simulink model "modelZSBmex"  (Simulink 8.3)
settings: Solver=ode4  StartTime=0.0  StopTime=0.2  FixedStep=0.01  RelTol=1e-3
settings Model: Creator=Chan Hwaiwing  LastModifiedBy=shubo
settings DataIOCC: SignalLoggingSaveFormat=Dataset
settings OptimizationCC: OptimizeModelRefInitCode=on  LifeSpan=1
settings DebuggingCC: UnderspecifiedInitializationDetection=Simplified  MergeDetectMultiDrivingBlocksExec=error  FrameProcessingCompatibilityMsg=error  StateNameClashWarn=none
settings RTWCC: SystemTargetFile=ert.tlc  TemplateMakefile=ert_default_tmf  Description=Embedded Coder  ProcessScript=ert_make_rtw_hook  BuildConfiguration=Faster Runs
settings CodeAppCC: IgnoreCustomStorageClasses=off
settings ERTTargetCC: MultiwordLength=2048  GenerateSampleERTMain=on  SupportNonFinite=off  SupportComplex=off  SupportContinuousTime=on  ERTCustomFileTemplate=example_file_process.tlc  ConvertIfToSwitch=off  SuppressUnreachableDefaultCases=off
settings ConfigComp: CovCompData="CovMetricSettings\t  dw"  CovFilter=CovHTMLOptions  CovHtmlReporting=on  CovSaveCumulativeToWorkspaceVar=on  CovSaveSingleToWorkspaceVar=on  CovModelRefExcluded="CovExternalEMLEnable\t  off"  CovSFcnEnable=off

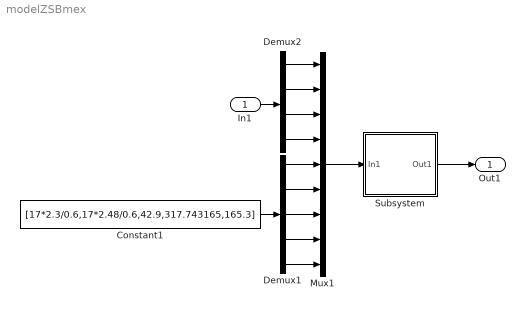
== system modelZSBmex ==
  In1 : Inport
  Constant1 : Constant  Value=[17*2.3/0.6,17*2.48/0.6,42.9,317.743165,165.3]
  Demux1 : Demux  Outputs=5
  Demux2 : Demux
  Mux1 : Mux  Inputs=9
  Subsystem : Subsystem
  Out1 : Outport
  wires:
  Subsystem/1(Out1) -> Out1/1
  Demux2/2 -> Mux1/2
  Demux2/4 -> Mux1/4
  Demux2/3 -> Mux1/3
  Demux2/1 -> Mux1/1
  Mux1/1 -> Subsystem/1(In1)
  In1/1 -> Demux2/1
  Constant1/1 -> Demux1/1
  Demux1/5 -> Mux1/9
  Demux1/2 -> Mux1/6
  Demux1/3 -> Mux1/7
  Demux1/4 -> Mux1/8
  Demux1/1 -> Mux1/5

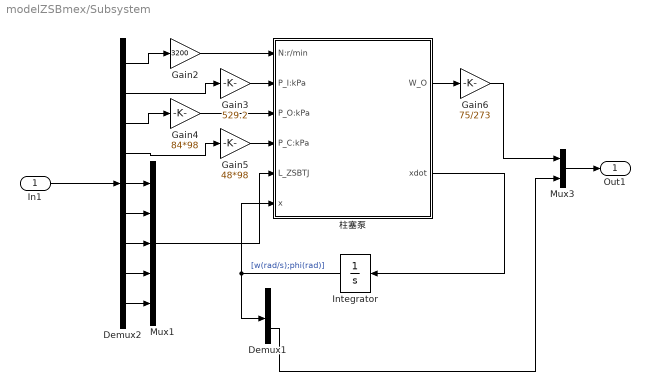
== system modelZSBmex/Subsystem ==
  In1 : Inport
  Demux1 : Demux  Outputs=2
  Demux2 : Demux  Outputs=9
  Gain2 : Gain  Gain=3200
  Gain3 : Gain  Gain=529.2
  Gain4 : Gain  Gain=84*98
  Gain5 : Gain  Gain=48*98
  Gain6 : Gain  Gain=75/273
  Integrator : Integrator  LimitOutput=on  UpperSaturationLimit=[999999 14.8/180*pi]  LowerSaturationLimit=[-999999 -0/180*pi ]
  Mux1 : Mux  Inputs=5
  Mux3 : Mux  Inputs=2
  柱塞泵 : Subsystem  AncestorBlock=HMMtoolbox/泵类/ZSB  mask(柱塞泵){L_ZSBHX=15, D_ZSBZS=48*2, A_ZSBZS=23.8*23.8*pi/4, RHO=780, ETA_V=0.95, M_ZS=0.1006, Z_ZSBZS=7, BETA_ZSBZS=12/180*pi, A_ZSBTJ=[pi*(33.26^2-17^2)/4, pi*(33.26^2-19.8^2)/4], L_ZSBTJ=[45 70 44 319 167], k=((1421-754.6)/((139.7-101.9)-(139.7-119.6))+(1754-1313)/((158-96.8)-(158-114.6)))*1e3*0.4, BETA_ZSBSD=6.97/180*pi, L_x0=139.7+85, J_ZSBXP=0.34*0.05, KD=7.65*0.5}
      mask prompts: L_ZSBHX "L_HX(等效滑靴厚度mm)"; D_ZSBZS "D_ZS(柱塞轴线在缸体的分布圆直径mm)"; A_ZSBZS "A_ZS(柱塞截面面积mm^2)"; RHO "RHO(标准状态下，油液密度kg/m^3)"; ETA_V "ETA_V(容积效率)"; M_ZS "M_ZS(柱塞质量)"; Z_ZSBZS "Z_ZS(柱塞数量)"; BETA_ZSBZS "BETA_ZS(柱塞安装角rad)"; A_ZSBTJ "A_TJ(面积参数向量mm^2)"; L_ZSBTJ "L_TJ(距离参数向量mm)"; k "k(弹簧弹性模量N/m)"; BETA_ZSBSD "BETA_SD(随动活塞安装角rad)"; L_x0 "L_x0(随动活塞初始位置mm)"; J_ZSBXP "J_XP(斜盘绕斜盘轴的转动惯量kg·m^2)"; KD "KD(斜盘转动阻力系数N·m·s/rad)"
      mask DialogControl DescTextVar Prompt: 填入相关参数
  Out1 : Outport
  wires:
  Gain2/1 -> 柱塞泵/1(N:r/min)
  Demux2/3 -> Gain4/1
  Mux3/1 -> Out1/1
  Gain3/1 -> 柱塞泵/2(P_I:kPa)
  In1/1 -> Demux2/1
  Integrator/1 -> Demux1/1, 柱塞泵/6(x)  "[w(rad/s);phi(rad)]"
  Demux2/2 -> Gain3/1
  Demux2/4 -> Gain5/1
  Demux2/1 -> Gain2/1
  柱塞泵/2(xdot) -> Integrator/1
  Mux1/1 -> 柱塞泵/5(L_ZSBTJ)
  柱塞泵/1(W_O) -> Gain6/1
  Gain6/1 -> Mux3/1
  Demux1/2 -> Mux3/2
  Gain4/1 -> 柱塞泵/3(P_O:kPa)
  Gain5/1 -> 柱塞泵/4(P_C:kPa)
  Demux2/5 -> Mux1/1
  Demux2/6 -> Mux1/2
  Demux2/9 -> Mux1/5
  Demux2/8 -> Mux1/4
  Demux2/7 -> Mux1/3

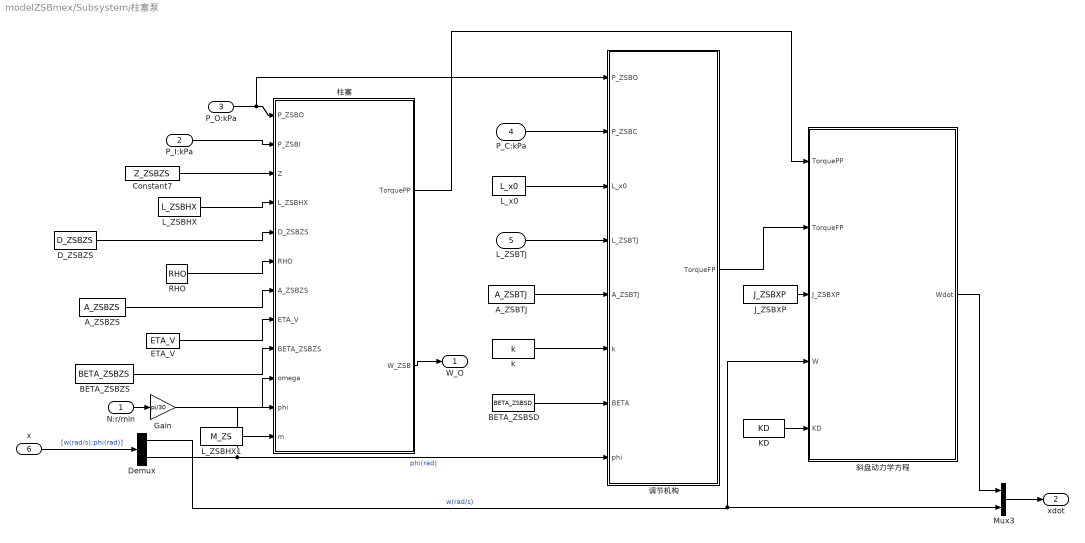
== system modelZSBmex/Subsystem/柱塞泵 ==
  N:r/min : Inport
  P_I:kPa : Inport  Port=2
  P_O:kPa : Inport  Port=3
  P_C:kPa : Inport  Port=4
  L_ZSBTJ : Inport  Port=5
  x : Inport  Port=6
  A_ZSBTJ : Constant  Value=A_ZSBTJ
  A_ZSBZS : Constant  Value=A_ZSBZS
  BETA_ZSBSD : Constant  Value=BETA_ZSBSD
  BETA_ZSBZS : Constant  Value=BETA_ZSBZS
  Constant7 : Constant  Value=Z_ZSBZS
  D_ZSBZS : Constant  Value=D_ZSBZS
  Demux : Demux  Outputs=2
  ETA_V : Constant  Value=ETA_V
  Gain : Gain  Gain=pi/30
  J_ZSBXP : Constant  Value=J_ZSBXP
  KD : Constant  Value=KD
  L_ZSBHX : Constant  Value=L_ZSBHX
  L_ZSBHX1 : Constant  Value=M_ZS
  L_x0 : Constant  Value=L_x0
  Mux3 : Mux  Inputs=2
  RHO : Constant  Value=RHO
  k : Constant  Value=k
  斜盘动力学方程 : MATLAB Function  TreatAsAtomicUnit=on
  柱塞 : MATLAB Function  TreatAsAtomicUnit=on
  调节机构 : MATLAB Function  TreatAsAtomicUnit=on
  W_O : Outport
  xdot : Outport  Port=2
  wires:
  x/1 -> Demux/1  "[w(rad/s);phi(rad)]"
  斜盘动力学方程/1(Wdot) -> Mux3/1
  Mux3/1 -> xdot/1
  J_ZSBXP/1 -> 斜盘动力学方程/3(J_ZSBXP)
  A_ZSBTJ/1 -> 调节机构/5(A_ZSBTJ)
  BETA_ZSBZS/1 -> 柱塞/9(BETA_ZSBZS)
  ETA_V/1 -> 柱塞/8(ETA_V)
  D_ZSBZS/1 -> 柱塞/5(D_ZSBZS)
  Demux/1 -> 斜盘动力学方程/4(W), Mux3/2  "w(rad/s)"
  柱塞/2(W_ZSB) -> W_O/1
  k/1 -> 调节机构/6(k)
  柱塞/1(TorquePP) -> 斜盘动力学方程/1(TorquePP)
  L_x0/1 -> 调节机构/3(L_x0)
  Gain/1 -> 柱塞/10(omega)
  BETA_ZSBSD/1 -> 调节机构/7(BETA)
  P_O:kPa/1 -> 调节机构/1(P_ZSBO), 柱塞/1(P_ZSBO)
  L_ZSBHX/1 -> 柱塞/4(L_ZSBHX)
  RHO/1 -> 柱塞/6(RHO)
  Constant7/1 -> 柱塞/3(Z)
  A_ZSBZS/1 -> 柱塞/7(A_ZSBZS)
  N:r/min/1 -> Gain/1
  Demux/2 -> 调节机构/8(phi), 柱塞/11(phi)  "phi(rad)"
  P_C:kPa/1 -> 调节机构/2(P_ZSBC)
  P_I:kPa/1 -> 柱塞/2(P_ZSBI)
  调节机构/1(TorqueFP) -> 斜盘动力学方程/2(TorqueFP)
  KD/1 -> 斜盘动力学方程/5(KD)
  L_ZSBTJ/1 -> 调节机构/4(L_ZSBTJ)
  L_ZSBHX1/1 -> 柱塞/12(m)

== matlab function Subsystem/柱塞泵/柱塞 ==
  data: P_ZSBO input double; P_ZSBI input double; Z input double; L_ZSBHX input double; D_ZSBZS input double; RHO input double; A_ZSBZS input double; ETA_V input double; BETA_ZSBZS input double; omega input double; TorquePP output double; W_ZSB output double; phi input double; m input double
function [ TorquePP, W_ZSB ] = Plunger_Pump(P_ZSBO,  P_ZSBI,  Z, L_ZSBHX, D_ZSBZS, RHO, A_ZSBZS, ETA_V,BETA_ZSBZS,omega,phi, m )

r=D_ZSBZS/2;
S_max = 2 * r * tan( phi );

TorqueLG = 0.5*r*r*Z*m*tan(phi)*omega*omega/cos(phi);
TorqueYY = -0.5*Z*L_ZSBHX*tan(phi)*A_ZSBZS*(P_ZSBO+P_ZSBI)/cos(phi);
TorquePP = (TorqueYY + TorqueLG) * 1e-6;

%-- Calculate q_tab and total Q --
W_ZSB = RHO * ETA_V *cos(BETA_ZSBZS)* A_ZSBZS * S_max * Z * omega * 0.5 / pi * 1e-9;

end

== matlab function Subsystem/柱塞泵/调节机构 ==
  data: P_ZSBO input double; TorqueFP output double; P_ZSBC input double; L_x0 input double; L_ZSBTJ input double; A_ZSBTJ input double; k input double; BETA input double; phi input double
function TorqueFP= TJ( P_ZSBO, P_ZSBC, L_x0, L_ZSBTJ, A_ZSBTJ, k, BETA, phi)

%计算活塞位置
xp = L_ZSBTJ(4)+L_ZSBTJ(1)*sin(phi+BETA)-L_ZSBTJ(5)-sqrt(L_ZSBTJ(3)*L_ZSBTJ(3)-(L_ZSBTJ(2)-L_ZSBTJ(1)*cos(phi+BETA))^2);

%计算随动活塞杆上的作用力
Pleft = P_ZSBO * 1e3;%kPa
Pright = Pleft-P_ZSBC * 1e3;%kPa
Fleft = Pleft * A_ZSBTJ(1) * 1e-6;%N
Fright = Pright * A_ZSBTJ(2) * 1e-6;%N
Fs = k * (L_x0 - xp) * 1e-3;
Fsui = Fs + Fright - Fleft;

%计算随动活塞杆力对斜盘作用力矩
delta = asin((L_ZSBTJ(2)-L_ZSBTJ(1)*cos(phi+BETA))/L_ZSBTJ(3));
TorqueFP = Fsui/cos(delta)*cos(delta-phi-BETA)*L_ZSBTJ(1)*1e-3;

end

== matlab function Subsystem/柱塞泵/斜盘动力学方程 ==
  data: TorquePP input double; Wdot output double; TorqueFP input double; J_ZSBXP input double; W input double; KD input double
function Wdot = DL(TorquePP,TorqueFP,J_ZSBXP,W, KD) 

    Torq_Net = TorquePP + TorqueFP - W * KD;
    Wdot =  Torq_Net / J_ZSBXP;
end
